simulink model "lab4task2"  (R2021a)
settings: Solver=VariableStepAuto  StartTime=0.0  StopTime=10.0  RelTol=1e-3
settings Model: Creator=Safi Ullah  LastModifiedBy=Safi Ullah

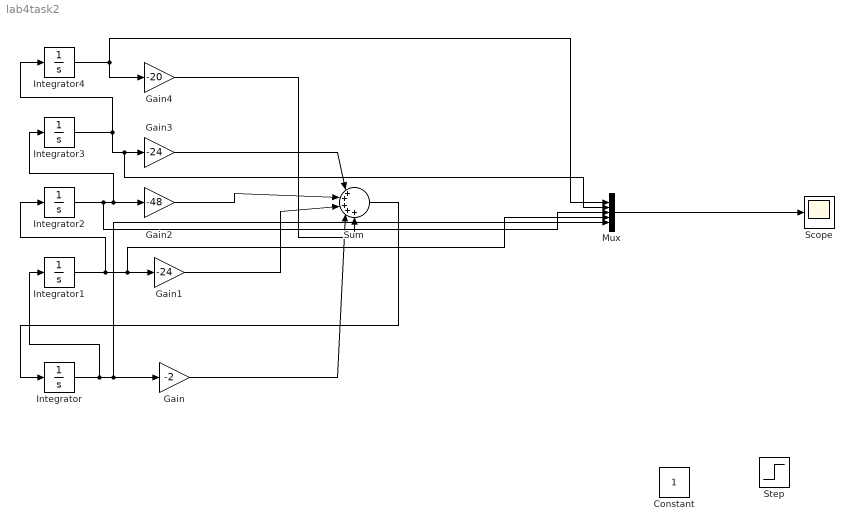
== system lab4task2 ==
  Constant : Constant
  Gain : Gain  Gain=-2
  Gain1 : Gain  Gain=-24
  Gain2 : Gain  Gain=-48
  Gain3 : Gain  Gain=-24
  Gain4 : Gain  Gain=-20
  Integrator : Integrator  InitialCondition=-7
  Integrator1 : Integrator  InitialCondition=-4
  Integrator2 : Integrator  InitialCondition=10
  Integrator3 : Integrator  InitialCondition=5
  Integrator4 : Integrator  InitialCondition=2
  Mux : Mux  Inputs=5
  Scope : Scope
  Step : Step  SampleTime=0
  Sum : Sum  Inputs=|+++++
  wires:
  Integrator/1 -> Integrator1/1, Mux/5, Gain/1
  Sum/1 -> Integrator/1
  Integrator1/1 -> Integrator2/1, Mux/4, Gain1/1
  Gain1/1 -> Sum/3
  Integrator2/1 -> Mux/3, Integrator3/1, Gain2/1
  Gain2/1 -> Sum/2
  Integrator3/1 -> Integrator4/1, Mux/2, Gain3/1
  Gain3/1 -> Sum/1
  Integrator4/1 -> Gain4/1, Mux/1
  Gain4/1 -> Sum/5
  Gain/1 -> Sum/4
  Mux/1 -> Scope/1
